simulink model "MPC_de_referencia_Sim"  (R2019b)
settings: Solver=VariableStepAuto  StartTime=0.0  StopTime=Tsim  RelTol=1e-3
libraries: cstblocks x2, mpclib x2
settings Model: Creator=victo  LastModifiedBy=victo
settings DataIOCC: ReturnWorkspaceOutputs=off
settings DebuggingCC: ArithmeticOperatorsInVariantConditions=warning
settings SFSimCC: SimUseLocalCustomCode=off  CustomCodeUndefinedFunction=UseInterfaceOnly
settings RTWCC: RTWUseLocalCustomCode=off
settings CodeAppCC: StateflowObjectComments=on

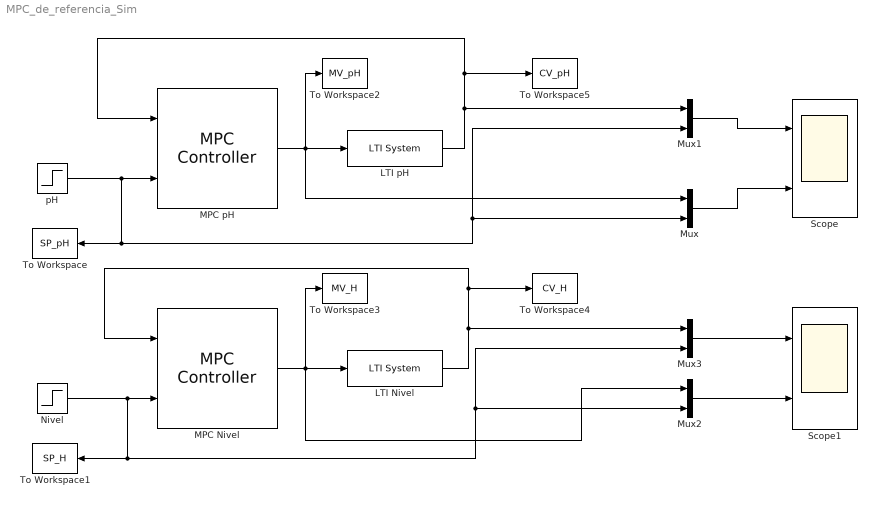
== system MPC_de_referencia_Sim ==
  LTI Nivel : cstblocks/LTI System  sys=Modelo_NIVEL  IC=[]
  LTI pH : cstblocks/LTI System  sys=Modelo_PH  IC=[]
  MPC Nivel : mpclib/MPC Controller  SCDEnableBlockLinearizationSpecification=on  mpcobj=mpcNivel_VD  is_multiple=0  enable_value=0  return_u0=off  updateMPCinCallerWorkspace=on  md_inport=off  mv_inport=off  uref_inport=off  return_cost=off  return_mvseq=off  return_qpstatus=off  return_xseq=off  return_state=off  return_ovseq=off  state_inport=off  umin_inport=off  umax_inport=off  ymin_inport=off  ymax_inport=off  cc_inport=off  ywt_inport=off  uwt_inport=off  duwt_inport=off  rhoeps_inport=off  pm_inport=off  MaximumP=10  HorizonChoice=FixedHorizon  n_ts=60  n_p=60  n_mv=1  n_md=0  n_ud=0  n_mo=1  n_uo=0  BlockDataType=double  SampleTimeInherited=off  switch_inport=off
  MPC pH : mpclib/MPC Controller  SCDEnableBlockLinearizationSpecification=on  mpcobj=mpcpH_VD  is_multiple=0  enable_value=0  return_u0=off  updateMPCinCallerWorkspace=on  md_inport=off  mv_inport=off  uref_inport=off  return_cost=off  return_mvseq=off  return_qpstatus=off  return_xseq=off  return_state=off  return_ovseq=off  state_inport=off  umin_inport=off  umax_inport=off  ymin_inport=off  ymax_inport=off  cc_inport=off  ywt_inport=off  uwt_inport=off  duwt_inport=off  rhoeps_inport=off  pm_inport=off  MaximumP=10  HorizonChoice=FixedHorizon  n_ts=60  n_p=60  n_mv=1  n_md=0  n_ud=0  n_mo=1  n_uo=0  BlockDataType=double  SampleTimeInherited=off  switch_inport=off
  Mux{,1..3} (4 alike) : Mux  Inputs=2
  Nivel : Step  Time=5000  Before=65  After=70  SampleTime=0
  Scope : Scope  NumInputPorts=2
  Scope1 : Scope  NumInputPorts=2
  To Workspace : ToWorkspace  VariableName=SP_pH  SampleTime=1
  To Workspace1 : ToWorkspace  VariableName=SP_H  SampleTime=1
  To Workspace2 : ToWorkspace  VariableName=MV_pH  SampleTime=1
  To Workspace3 : ToWorkspace  VariableName=MV_H  SampleTime=1
  To Workspace4 : ToWorkspace  VariableName=CV_H  SampleTime=1
  To Workspace5 : ToWorkspace  VariableName=CV_pH  SampleTime=1
  pH : Step  Time=5000  Before=7  After=7.5  SampleTime=0
  wires:
  MPC pH/1 -> To Workspace2/1, Mux/1, LTI pH/1
  LTI pH/1 -> Mux1/1, To Workspace5/1, MPC pH/1
  MPC Nivel/1 -> To Workspace3/1, Mux2/1, LTI Nivel/1
  LTI Nivel/1 -> Mux3/1, MPC Nivel/1, To Workspace4/1
  Mux1/1 -> Scope/1
  Mux/1 -> Scope/2
  Mux2/1 -> Scope1/2
  Mux3/1 -> Scope1/1
  pH/1 -> To Workspace/1, Mux1/2, Mux/2, MPC pH/2
  Nivel/1 -> To Workspace1/1, Mux3/2, Mux2/2, MPC Nivel/2
